simulink model "Simulation"  (R2023b)
settings: Solver=VariableStepAuto  StartTime=0.0  StopTime=2  RelTol=1e-3
InitFcn:
  | Tsc=0.0001;
  | Rs=0.0113929;
  | Rr=0.0197883;
  | Ls=0.007145;
  | Lr=0.007145;
  | Lm=0.007045;
  | w_c=100;
libraries: slpidlib x6, simulink x1, spspowerguiLib x1
(part 1 of 2)
settings Model: Creator=zugzh  LastModifiedBy=zugzh
settings DebuggingCC: IgnoredZcDiagnostic=none

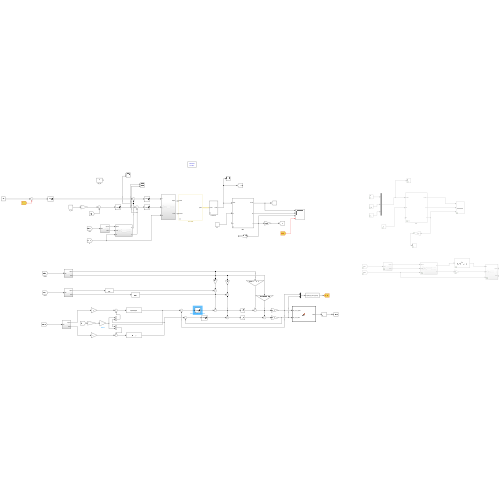
[thumbnail: Simulink's stored preview of the top-level diagram]
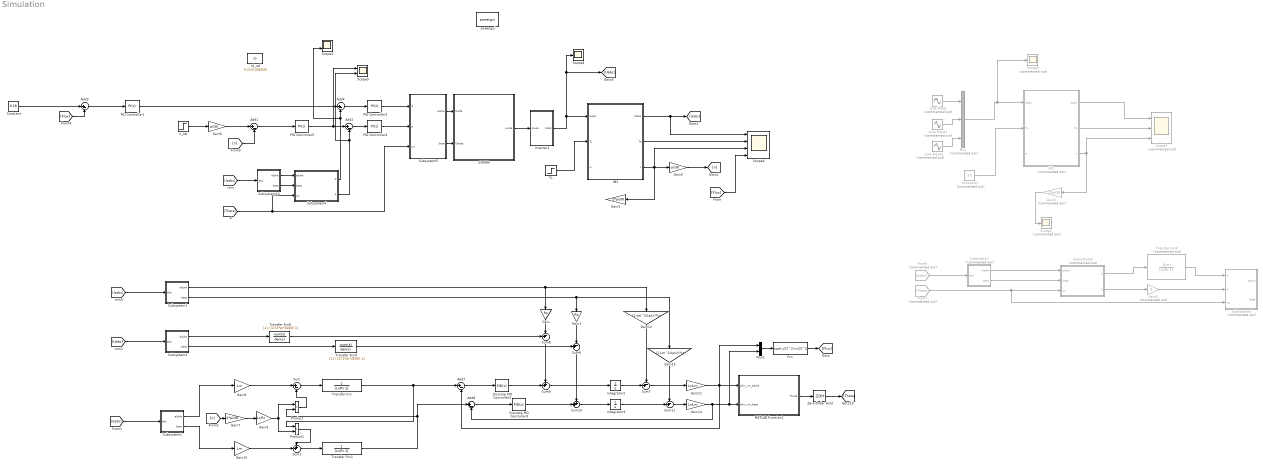
== system Simulation ==
  Add{1..4,7..8} (6 alike) : Sum  Inputs=|+-
  Constant : Constant  Value=0.18
  Constant1 : Constant  Commented=on  Value=75
  Discrete PID Controller2 : slpidlib/PID Controller  Controller=PID  Form=Parallel  TimeDomain=Discrete-time  UseExternalTs=off  SampleTime=-1  IntegratorMethod=Forward Euler  FilterMethod=Forward Euler  ControllerParametersSource=internal  P=sqrt(2)*w_c  I=w_c^2  UseKiTs=off  D=0  N=100  UseFilter=on  TunerSelectOption=Transfer Function Based (PID Tuner App)  InitialConditionSource=internal  InitialConditionForIntegrator=0  InitialConditionForFilter=0  DifferentiatorICPrevScaledInput=0  ExternalReset=none  TrackingMode=off  Kt=1  LimitOutput=on  SatLimitsSource=internal  UpperSaturationLimit=340  LowerSaturationLimit=-340  LinearizeAsGain=off  AntiWindupMode=none  Kb=1  LimitIntegrator=off  UpperIntegratorSaturationLimit=inf  LowerIntegratorSaturationLimit=-inf  POutMin=[]  POutMax=[]  IOutMin=[]  IOutMax=[]  DOutMin=[]  DOutMax=[]  NOutMin=[]  NOutMax=[]  SumOutMin=[]  SumOutMax=[]  SaturationOutMin=[]  SaturationOutMax=[]  PParamMin=[]  PParamMax=[]  IParamMin=[]  IParamMax=[]  DParamMin=[]  DParamMax=[]  NParamMin=[]  NParamMax=[]  KbParamMin=[]  KbParamMax=[]  KtParamMin=[]  KtParamMax=[]  KbOutMin=[]  KbOutMax=[]  KtOutMin=[]  KtOutMax=[]  IntegratorOutMin=[]  IntegratorOutMax=[]  FilterOutMin=[]  FilterOutMax=[]  SumI1OutMin=[]  SumI1OutMax=[]  SumI2OutMin=[]  SumI2OutMax=[]  SumI3OutMin=[]  SumI3OutMax=[]  SumI4OutMin=[]  SumI4OutMax=[]  SumDOutMin=[]  SumDOutMax=[]  DifferentiatorOutMin=[]  DifferentiatorOutMax=[]  FilterDiffOutCoefMin=[]  FilterDiffOutCoefMax=[]  ReciprocalOutMin=[]  ReciprocalOutMax=[]  SumDenOutMin=[]  SumDenOutMax=[]  SumNumOutMin=[]  SumNumOutMax=[]  DivideOutMin=[]  DivideOutMax=[]  UdiffTsProdOutMin=[]  UdiffTsProdOutMax=[]  NTsProdOutMin=[]  NTsProdOutMax=[]  UintegralTsProdOutMin=[]  UintegralTsProdOutMax=[]  UngainTsProdOutMin=[]  UngainTsProdOutMax=[]  ClampingZeroOutDataTypeStr=Inherit: Inherit via back propagation  ClampingZeroOutMin=[]  ClampingZeroOutMax=[]  FilterDenConstantOutDataTypeStr=Inherit: Inherit via back propagation  FilterDenConstantOutMin=[]  FilterDenConstantOutMax=[]  PCopyOutDataTypeStr=Inherit: Inherit via back propagation  PCopyOutMin=[]  PCopyOutMax=[]  NCopyOutDataTypeStr=Inherit: Inherit via back propagation  NCopyOutMin=[]  NCopyOutMax=[]  IntegratorContinuousStateAttributes=''  IntegratorStateMustResolveToSignalObject=off  IntegratorRTWStateStorageClass=Auto  FilterContinuousStateAttributes=''  FilterStateMustResolveToSignalObject=off  FilterRTWStateStorageClass=Auto  ParallelPVariant=InternalParameters  IdealPVariant=Disabled  IVariant=InternalParameters  DVariant=InternalParameters  IntegratorVariant=Discrete  SatVariant=Enabled  AWVariant=Passthrough  PCopyVariant=Disabled  TRVariant=Disabled  FdbkBlocksVariant=Forward  IdealPFdbkVariant=Disabled  SatFdbkVariant=Disabled  DerivativeFilterVariant=ForwardEulerFilter  NVariant=InternalParameters  NCopyVariant=Disabled  FilterICVariant=InternalICsFilter  IntegratorICVariant=InternalICs  ExternalResetVariant=Disabled  TRSumVariant=Passthrough  SumFdbkVariant=Disabled  SumVariant=Sum_PID  TsampFilterVariant=InternalTs  TsampNgainVariant=Passthrough  TsampIntegralVariant=Disabled_SignalSpec  ExternalSaturationOutDataTypeStr=Inherit: Same as second input
      settings: LibrarySourceBlock=hdlsllib/Discrete/Discrete PID Controller
  Discrete PID Controller3 : slpidlib/PID Controller  Controller=PID  Form=Parallel  TimeDomain=Discrete-time  UseExternalTs=off  SampleTime=-1  IntegratorMethod=Forward Euler  FilterMethod=Forward Euler  ControllerParametersSource=internal  P=sqrt(2)*w_c  I=w_c^2  UseKiTs=off  D=0  N=100  UseFilter=on  TunerSelectOption=Transfer Function Based (PID Tuner App)  InitialConditionSource=internal  InitialConditionForIntegrator=0  InitialConditionForFilter=0  DifferentiatorICPrevScaledInput=0  ExternalReset=none  TrackingMode=off  Kt=1  LimitOutput=on  SatLimitsSource=internal  UpperSaturationLimit=340  LowerSaturationLimit=-340  LinearizeAsGain=off  AntiWindupMode=none  Kb=1  LimitIntegrator=off  UpperIntegratorSaturationLimit=inf  LowerIntegratorSaturationLimit=-inf  POutMin=[]  POutMax=[]  IOutMin=[]  IOutMax=[]  DOutMin=[]  DOutMax=[]  NOutMin=[]  NOutMax=[]  SumOutMin=[]  SumOutMax=[]  SaturationOutMin=[]  SaturationOutMax=[]  PParamMin=[]  PParamMax=[]  IParamMin=[]  IParamMax=[]  DParamMin=[]  DParamMax=[]  NParamMin=[]  NParamMax=[]  KbParamMin=[]  KbParamMax=[]  KtParamMin=[]  KtParamMax=[]  KbOutMin=[]  KbOutMax=[]  KtOutMin=[]  KtOutMax=[]  IntegratorOutMin=[]  IntegratorOutMax=[]  FilterOutMin=[]  FilterOutMax=[]  SumI1OutMin=[]  SumI1OutMax=[]  SumI2OutMin=[]  SumI2OutMax=[]  SumI3OutMin=[]  SumI3OutMax=[]  SumI4OutMin=[]  SumI4OutMax=[]  SumDOutMin=[]  SumDOutMax=[]  DifferentiatorOutMin=[]  DifferentiatorOutMax=[]  FilterDiffOutCoefMin=[]  FilterDiffOutCoefMax=[]  ReciprocalOutMin=[]  ReciprocalOutMax=[]  SumDenOutMin=[]  SumDenOutMax=[]  SumNumOutMin=[]  SumNumOutMax=[]  DivideOutMin=[]  DivideOutMax=[]  UdiffTsProdOutMin=[]  UdiffTsProdOutMax=[]  NTsProdOutMin=[]  NTsProdOutMax=[]  UintegralTsProdOutMin=[]  UintegralTsProdOutMax=[]  UngainTsProdOutMin=[]  UngainTsProdOutMax=[]  ClampingZeroOutDataTypeStr=Inherit: Inherit via back propagation  ClampingZeroOutMin=[]  ClampingZeroOutMax=[]  FilterDenConstantOutDataTypeStr=Inherit: Inherit via back propagation  FilterDenConstantOutMin=[]  FilterDenConstantOutMax=[]  PCopyOutDataTypeStr=Inherit: Inherit via back propagation  PCopyOutMin=[]  PCopyOutMax=[]  NCopyOutDataTypeStr=Inherit: Inherit via back propagation  NCopyOutMin=[]  NCopyOutMax=[]  IntegratorContinuousStateAttributes=''  IntegratorStateMustResolveToSignalObject=off  IntegratorRTWStateStorageClass=Auto  FilterContinuousStateAttributes=''  FilterStateMustResolveToSignalObject=off  FilterRTWStateStorageClass=Auto  ParallelPVariant=InternalParameters  IdealPVariant=Disabled  IVariant=InternalParameters  DVariant=InternalParameters  IntegratorVariant=Discrete  SatVariant=Enabled  AWVariant=Passthrough  PCopyVariant=Disabled  TRVariant=Disabled  FdbkBlocksVariant=Forward  IdealPFdbkVariant=Disabled  SatFdbkVariant=Disabled  DerivativeFilterVariant=ForwardEulerFilter  NVariant=InternalParameters  NCopyVariant=Disabled  FilterICVariant=InternalICsFilter  IntegratorICVariant=InternalICs  ExternalResetVariant=Disabled  TRSumVariant=Passthrough  SumFdbkVariant=Disabled  SumVariant=Sum_PID  TsampFilterVariant=InternalTs  TsampNgainVariant=Passthrough  TsampIntegralVariant=Disabled_SignalSpec  ExternalSaturationOutDataTypeStr=Inherit: Same as second input
      settings: LibrarySourceBlock=hdlsllib/Discrete/Discrete PID Controller
  Fcn : Fcn  Expr=sqrt(u(1)^2+u(2)^2)
  From6 : From  Commented=on  GotoTag=Isabc
  From7 : From  Commented=on  GotoTag=Theta
  Gain : Gain  Gain=Rs
  Gain1 : Gain  Gain=Rs
  Gain10 : Gain  Gain=Lm
  Gain11 : Gain  Gain=Lr/Lm
  Gain12 : Gain  Gain=(1-Lm^2/Ls/Lr)*Ls
  Gain14 : Gain  Gain=Lr/Lm
  Gain15 : Gain  Gain=(1-Lm^2/Ls/Lr)*Ls
  Gain2 : Gain  Commented=on  Gain=2*pi/30
  Gain3 : Gain  Gain=2*pi/30
  Gain4 : Gain  Commented=on  Gain=0
  Gain5 : Gain  Gain=pi/30
  Gain6 : Gain  Gain=pi/30
  Gain7 : Gain  Gain=2*pi/30
  Gain8 : Gain  Gain=Lm
  Gain9 : Gain  Gain=Lr/Rr
  IM1 : Subsystem  Commented=on  mask{Rs=0.0113929, Rr=0.0197883, Ls=0.006145, Lr=0.006145, Lm=0.006045, J=0.0952384, np=2}
      mask prompts: Rs "Rs(Ohm)"; Rr "Rr(Ohm)"; Ls "Ls(H)"; Lr "Lr(H)"; Lm "Lm(H)"; J "J(kg*m^2)"; np "Np()"
  IM2 : Subsystem  mask{Rs=0.0113929, Rr=0.0197883, Ls=0.007145, Lr=0.007145, Lm=0.007045, J=0.0952384, np=2}
      mask prompts: Rs "Rs(Ohm)"; Rr "Rr(Ohm)"; Ls "Ls(H)"; Lr "Lr(H)"; Lm "Lm(H)"; J "J(kg*m^2)"; np "Np()"
  Id_ref : Constant  Value=0.21/0.006045
  Integrator2 : Integrator  InitialCondition=0.001  LimitOutput=on  UpperSaturationLimit=1e6  LowerSaturationLimit=-1e6
  Integrator3 : Integrator  InitialCondition=0.001  LimitOutput=on  UpperSaturationLimit=1e6  LowerSaturationLimit=-1e6
  Inverter1 : Subsystem  mask(Inverter){Udc=540}
      mask prompts: Udc "Udc(V)"
  MATLAB Function1 : MATLAB Function  TreatAsAtomicUnit=on
  Mux : Mux  Commented=on  Inputs=3
  Mux1 : Mux  Inputs=2
  PID Controller1 : slpidlib/PID Controller  Controller=PI  Form=Parallel  TimeDomain=Discrete-time  UseExternalTs=off  SampleTime=-1  IntegratorMethod=Forward Euler  FilterMethod=Forward Euler  ControllerParametersSource=internal  P=1000  I=4000  UseKiTs=off  D=1  N=100  UseFilter=on  TunerSelectOption=Transfer Function Based (PID Tuner App)  InitialConditionSource=internal  InitialConditionForIntegrator=0  InitialConditionForFilter=0  DifferentiatorICPrevScaledInput=0  ExternalReset=none  TrackingMode=off  Kt=1  LimitOutput=on  SatLimitsSource=internal  UpperSaturationLimit=340  LowerSaturationLimit=-340  LinearizeAsGain=on  AntiWindupMode=none  Kb=1  LimitIntegrator=off  UpperIntegratorSaturationLimit=inf  LowerIntegratorSaturationLimit=-inf  POutMin=[]  POutMax=[]  IOutMin=[]  IOutMax=[]  DOutMin=[]  DOutMax=[]  NOutMin=[]  NOutMax=[]  SumOutMin=[]  SumOutMax=[]  SaturationOutMin=[]  SaturationOutMax=[]  PParamMin=[]  PParamMax=[]  IParamMin=[]  IParamMax=[]  DParamMin=[]  DParamMax=[]  NParamMin=[]  NParamMax=[]  KbParamMin=[]  KbParamMax=[]  KtParamMin=[]  KtParamMax=[]  KbOutMin=[]  KbOutMax=[]  KtOutMin=[]  KtOutMax=[]  IntegratorOutMin=[]  IntegratorOutMax=[]  FilterOutMin=[]  FilterOutMax=[]  SumI1OutMin=[]  SumI1OutMax=[]  SumI2OutMin=[]  SumI2OutMax=[]  SumI3OutMin=[]  SumI3OutMax=[]  SumI4OutMin=[]  SumI4OutMax=[]  SumDOutMin=[]  SumDOutMax=[]  DifferentiatorOutMin=[]  DifferentiatorOutMax=[]  FilterDiffOutCoefMin=[]  FilterDiffOutCoefMax=[]  ReciprocalOutMin=[]  ReciprocalOutMax=[]  SumDenOutMin=[]  SumDenOutMax=[]  SumNumOutMin=[]  SumNumOutMax=[]  DivideOutMin=[]  DivideOutMax=[]  UdiffTsProdOutMin=[]  UdiffTsProdOutMax=[]  NTsProdOutMin=[]  NTsProdOutMax=[]  UintegralTsProdOutMin=[]  UintegralTsProdOutMax=[]  UngainTsProdOutMin=[]  UngainTsProdOutMax=[]  ClampingZeroOutDataTypeStr=Inherit: Inherit via back propagation  ClampingZeroOutMin=[]  ClampingZeroOutMax=[]  FilterDenConstantOutDataTypeStr=Inherit: Inherit via back propagation  FilterDenConstantOutMin=[]  FilterDenConstantOutMax=[]  PCopyOutDataTypeStr=Inherit: Inherit via back propagation  PCopyOutMin=[]  PCopyOutMax=[]  NCopyOutDataTypeStr=Inherit: Inherit via back propagation  NCopyOutMin=[]  NCopyOutMax=[]  IntegratorContinuousStateAttributes=''  IntegratorStateMustResolveToSignalObject=off  IntegratorRTWStateStorageClass=Auto  FilterContinuousStateAttributes=''  FilterStateMustResolveToSignalObject=off  FilterRTWStateStorageClass=Auto  ParallelPVariant=InternalParameters  IdealPVariant=Disabled  IVariant=InternalParameters  DVariant=Disabled  IntegratorVariant=Discrete  SatVariant=Enabled  AWVariant=Passthrough  PCopyVariant=Disabled  TRVariant=Disabled  FdbkBlocksVariant=Forward  IdealPFdbkVariant=Disabled  SatFdbkVariant=Disabled  DerivativeFilterVariant=Disabled  NVariant=Disabled  NCopyVariant=Disabled_SignalSpec  FilterICVariant=Disabled  IntegratorICVariant=InternalICs  ExternalResetVariant=Disabled  TRSumVariant=Passthrough  SumFdbkVariant=Disabled  SumVariant=Sum_PI  TsampFilterVariant=InternalTs  TsampNgainVariant=Passthrough  TsampIntegralVariant=Disabled_SignalSpec  ExternalSaturationOutDataTypeStr=Inherit: Same as second input
  PID Controller3 : slpidlib/PID Controller  Controller=PI  Form=Parallel  TimeDomain=Discrete-time  UseExternalTs=off  SampleTime=-1  IntegratorMethod=Forward Euler  FilterMethod=Forward Euler  ControllerParametersSource=internal  P=0.656736650875738  I=37.717571379892140  UseKiTs=off  D=1  N=100  UseFilter=on  TunerSelectOption=Transfer Function Based (PID Tuner App)  InitialConditionSource=internal  InitialConditionForIntegrator=0  InitialConditionForFilter=0  DifferentiatorICPrevScaledInput=0  ExternalReset=none  TrackingMode=off  Kt=1  LimitOutput=on  SatLimitsSource=internal  UpperSaturationLimit=340  LowerSaturationLimit=-340  LinearizeAsGain=on  AntiWindupMode=none  Kb=1  LimitIntegrator=off  UpperIntegratorSaturationLimit=inf  LowerIntegratorSaturationLimit=-inf  POutMin=[]  POutMax=[]  IOutMin=[]  IOutMax=[]  DOutMin=[]  DOutMax=[]  NOutMin=[]  NOutMax=[]  SumOutMin=[]  SumOutMax=[]  SaturationOutMin=[]  SaturationOutMax=[]  PParamMin=[]  PParamMax=[]  IParamMin=[]  IParamMax=[]  DParamMin=[]  DParamMax=[]  NParamMin=[]  NParamMax=[]  KbParamMin=[]  KbParamMax=[]  KtParamMin=[]  KtParamMax=[]  KbOutMin=[]  KbOutMax=[]  KtOutMin=[]  KtOutMax=[]  IntegratorOutMin=[]  IntegratorOutMax=[]  FilterOutMin=[]  FilterOutMax=[]  SumI1OutMin=[]  SumI1OutMax=[]  SumI2OutMin=[]  SumI2OutMax=[]  SumI3OutMin=[]  SumI3OutMax=[]  SumI4OutMin=[]  SumI4OutMax=[]  SumDOutMin=[]  SumDOutMax=[]  DifferentiatorOutMin=[]  DifferentiatorOutMax=[]  FilterDiffOutCoefMin=[]  FilterDiffOutCoefMax=[]  ReciprocalOutMin=[]  ReciprocalOutMax=[]  SumDenOutMin=[]  SumDenOutMax=[]  SumNumOutMin=[]  SumNumOutMax=[]  DivideOutMin=[]  DivideOutMax=[]  UdiffTsProdOutMin=[]  UdiffTsProdOutMax=[]  NTsProdOutMin=[]  NTsProdOutMax=[]  UintegralTsProdOutMin=[]  UintegralTsProdOutMax=[]  UngainTsProdOutMin=[]  UngainTsProdOutMax=[]  ClampingZeroOutDataTypeStr=Inherit: Inherit via back propagation  ClampingZeroOutMin=[]  ClampingZeroOutMax=[]  FilterDenConstantOutDataTypeStr=Inherit: Inherit via back propagation  FilterDenConstantOutMin=[]  FilterDenConstantOutMax=[]  PCopyOutDataTypeStr=Inherit: Inherit via back propagation  PCopyOutMin=[]  PCopyOutMax=[]  NCopyOutDataTypeStr=Inherit: Inherit via back propagation  NCopyOutMin=[]  NCopyOutMax=[]  IntegratorContinuousStateAttributes=''  IntegratorStateMustResolveToSignalObject=off  IntegratorRTWStateStorageClass=Auto  FilterContinuousStateAttributes=''  FilterStateMustResolveToSignalObject=off  FilterRTWStateStorageClass=Auto  ParallelPVariant=InternalParameters  IdealPVariant=Disabled  IVariant=InternalParameters  DVariant=Disabled  IntegratorVariant=Discrete  SatVariant=Enabled  AWVariant=Passthrough  PCopyVariant=Disabled  TRVariant=Disabled  FdbkBlocksVariant=Forward  IdealPFdbkVariant=Disabled  SatFdbkVariant=Disabled  DerivativeFilterVariant=Disabled  NVariant=Disabled  NCopyVariant=Disabled_SignalSpec  FilterICVariant=Disabled  IntegratorICVariant=InternalICs  ExternalResetVariant=Disabled  TRSumVariant=Passthrough  SumFdbkVariant=Disabled  SumVariant=Sum_PI  TsampFilterVariant=InternalTs  TsampNgainVariant=Passthrough  TsampIntegralVariant=Disabled_SignalSpec  ExternalSaturationOutDataTypeStr=Inherit: Same as second input
  PID Controller4 : slpidlib/PID Controller  Controller=PI  Form=Parallel  TimeDomain=Discrete-time  UseExternalTs=off  SampleTime=-1  IntegratorMethod=Forward Euler  FilterMethod=Forward Euler  ControllerParametersSource=internal  P=0.656736650875738  I=1.011142867406485e+02  UseKiTs=off  D=1  N=100  UseFilter=on  TunerSelectOption=Transfer Function Based (PID Tuner App)  InitialConditionSource=internal  InitialConditionForIntegrator=0  InitialConditionForFilter=0  DifferentiatorICPrevScaledInput=0  ExternalReset=none  TrackingMode=off  Kt=1  LimitOutput=on  SatLimitsSource=internal  UpperSaturationLimit=340  LowerSaturationLimit=-340  LinearizeAsGain=on  AntiWindupMode=none  Kb=1  LimitIntegrator=off  UpperIntegratorSaturationLimit=inf  LowerIntegratorSaturationLimit=-inf  POutMin=[]  POutMax=[]  IOutMin=[]  IOutMax=[]  DOutMin=[]  DOutMax=[]  NOutMin=[]  NOutMax=[]  SumOutMin=[]  SumOutMax=[]  SaturationOutMin=[]  SaturationOutMax=[]  PParamMin=[]  PParamMax=[]  IParamMin=[]  IParamMax=[]  DParamMin=[]  DParamMax=[]  NParamMin=[]  NParamMax=[]  KbParamMin=[]  KbParamMax=[]  KtParamMin=[]  KtParamMax=[]  KbOutMin=[]  KbOutMax=[]  KtOutMin=[]  KtOutMax=[]  IntegratorOutMin=[]  IntegratorOutMax=[]  FilterOutMin=[]  FilterOutMax=[]  SumI1OutMin=[]  SumI1OutMax=[]  SumI2OutMin=[]  SumI2OutMax=[]  SumI3OutMin=[]  SumI3OutMax=[]  SumI4OutMin=[]  SumI4OutMax=[]  SumDOutMin=[]  SumDOutMax=[]  DifferentiatorOutMin=[]  DifferentiatorOutMax=[]  FilterDiffOutCoefMin=[]  FilterDiffOutCoefMax=[]  ReciprocalOutMin=[]  ReciprocalOutMax=[]  SumDenOutMin=[]  SumDenOutMax=[]  SumNumOutMin=[]  SumNumOutMax=[]  DivideOutMin=[]  DivideOutMax=[]  UdiffTsProdOutMin=[]  UdiffTsProdOutMax=[]  NTsProdOutMin=[]  NTsProdOutMax=[]  UintegralTsProdOutMin=[]  UintegralTsProdOutMax=[]  UngainTsProdOutMin=[]  UngainTsProdOutMax=[]  ClampingZeroOutDataTypeStr=Inherit: Inherit via back propagation  ClampingZeroOutMin=[]  ClampingZeroOutMax=[]  FilterDenConstantOutDataTypeStr=Inherit: Inherit via back propagation  FilterDenConstantOutMin=[]  FilterDenConstantOutMax=[]  PCopyOutDataTypeStr=Inherit: Inherit via back propagation  PCopyOutMin=[]  PCopyOutMax=[]  NCopyOutDataTypeStr=Inherit: Inherit via back propagation  NCopyOutMin=[]  NCopyOutMax=[]  IntegratorContinuousStateAttributes=''  IntegratorStateMustResolveToSignalObject=off  IntegratorRTWStateStorageClass=Auto  FilterContinuousStateAttributes=''  FilterStateMustResolveToSignalObject=off  FilterRTWStateStorageClass=Auto  ParallelPVariant=InternalParameters  IdealPVariant=Disabled  IVariant=InternalParameters  DVariant=Disabled  IntegratorVariant=Discrete  SatVariant=Enabled  AWVariant=Passthrough  PCopyVariant=Disabled  TRVariant=Disabled  FdbkBlocksVariant=Forward  IdealPFdbkVariant=Disabled  SatFdbkVariant=Disabled  DerivativeFilterVariant=Disabled  NVariant=Disabled  NCopyVariant=Disabled_SignalSpec  FilterICVariant=Disabled  IntegratorICVariant=InternalICs  ExternalResetVariant=Disabled  TRSumVariant=Passthrough  SumFdbkVariant=Disabled  SumVariant=Sum_PI  TsampFilterVariant=InternalTs  TsampNgainVariant=Passthrough  TsampIntegralVariant=Disabled_SignalSpec  ExternalSaturationOutDataTypeStr=Inherit: Same as second input
  PID Controller5 : slpidlib/PID Controller  Controller=PI  Form=Parallel  TimeDomain=Discrete-time  UseExternalTs=off  SampleTime=Tsc  IntegratorMethod=Forward Euler  FilterMethod=Forward Euler  ControllerParametersSource=internal  P=2.769062140173488e+03  I=1.980890752650220e+06  UseKiTs=off  D=0  N=100  UseFilter=on  TunerSelectOption=Transfer Function Based (PID Tuner App)  InitialConditionSource=internal  InitialConditionForIntegrator=0  InitialConditionForFilter=0  DifferentiatorICPrevScaledInput=0  ExternalReset=none  TrackingMode=off  Kt=1  LimitOutput=on  SatLimitsSource=internal  UpperSaturationLimit=196  LowerSaturationLimit=-196  LinearizeAsGain=off  AntiWindupMode=clamping  Kb=1  LimitIntegrator=off  UpperIntegratorSaturationLimit=inf  LowerIntegratorSaturationLimit=-inf  POutMin=[]  POutMax=[]  IOutMin=[]  IOutMax=[]  DOutMin=[]  DOutMax=[]  NOutMin=[]  NOutMax=[]  SumOutMin=[]  SumOutMax=[]  SaturationOutMin=[]  SaturationOutMax=[]  PParamMin=[]  PParamMax=[]  IParamMin=[]  IParamMax=[]  DParamMin=[]  DParamMax=[]  NParamMin=[]  NParamMax=[]  KbParamMin=[]  KbParamMax=[]  KtParamMin=[]  KtParamMax=[]  KbOutMin=[]  KbOutMax=[]  KtOutMin=[]  KtOutMax=[]  IntegratorOutMin=[]  IntegratorOutMax=[]  FilterOutMin=[]  FilterOutMax=[]  SumI1OutMin=[]  SumI1OutMax=[]  SumI2OutMin=[]  SumI2OutMax=[]  SumI3OutMin=[]  SumI3OutMax=[]  SumI4OutMin=[]  SumI4OutMax=[]  SumDOutMin=[]  SumDOutMax=[]  DifferentiatorOutMin=[]  DifferentiatorOutMax=[]  FilterDiffOutCoefMin=[]  FilterDiffOutCoefMax=[]  ReciprocalOutMin=[]  ReciprocalOutMax=[]  SumDenOutMin=[]  SumDenOutMax=[]  SumNumOutMin=[]  SumNumOutMax=[]  DivideOutMin=[]  DivideOutMax=[]  UdiffTsProdOutMin=[]  UdiffTsProdOutMax=[]  NTsProdOutMin=[]  NTsProdOutMax=[]  UintegralTsProdOutMin=[]  UintegralTsProdOutMax=[]  UngainTsProdOutMin=[]  UngainTsProdOutMax=[]  ClampingZeroOutDataTypeStr=Inherit: Inherit via back propagation  ClampingZeroOutMin=[]  ClampingZeroOutMax=[]  FilterDenConstantOutDataTypeStr=Inherit: Inherit via back propagation  FilterDenConstantOutMin=[]  FilterDenConstantOutMax=[]  PCopyOutDataTypeStr=Inherit: Inherit via back propagation  PCopyOutMin=[]  PCopyOutMax=[]  NCopyOutDataTypeStr=Inherit: Inherit via back propagation  NCopyOutMin=[]  NCopyOutMax=[]  IntegratorContinuousStateAttributes=''  IntegratorStateMustResolveToSignalObject=off  IntegratorRTWStateStorageClass=Auto  FilterContinuousStateAttributes=''  FilterStateMustResolveToSignalObject=off  FilterRTWStateStorageClass=Auto  ParallelPVariant=InternalParameters  IdealPVariant=Disabled  IVariant=InternalParameters  DVariant=Disabled  IntegratorVariant=Discrete  SatVariant=Enabled  AWVariant=DiscClampingParallel  PCopyVariant=Disabled  TRVariant=Disabled  FdbkBlocksVariant=Forward  IdealPFdbkVariant=Disabled  SatFdbkVariant=Disabled  DerivativeFilterVariant=Disabled  NVariant=Disabled  NCopyVariant=Disabled_SignalSpec  FilterICVariant=Disabled  IntegratorICVariant=InternalICs  ExternalResetVariant=Disabled  TRSumVariant=Passthrough  SumFdbkVariant=Disabled  SumVariant=Sum_PI  TsampFilterVariant=InternalTs  TsampNgainVariant=Passthrough  TsampIntegralVariant=Disabled_SignalSpec  ExternalSaturationOutDataTypeStr=Inherit: Same as second input
  Product : Product
  Product1 : Product
  SVPWM : Subsystem  mask{Ts=1/10000, Udc=540}
  Scope1 : Scope  Commented=on
  Scope2 : Scope  NumInputPorts=2
  Scope3 : Scope  Commented=on  NumInputPorts=3
  Scope4 : Scope  NumInputPorts=4
  Scope5 : Scope  NumInputPorts=2
  Scope8 : Scope
  Scope9 : Scope  Commented=on
  Sine Wave : Sin  Commented=on  Amplitude=244.949  Frequency=4567.25/60*2*2*pi*(1+0.0425049)  SampleTime=0
  Sine Wave1 : Sin  Commented=on  Amplitude=244.949  Frequency=4567.25/60*2*2*pi*(1+0.0425049)  Phase=-2*pi/3  SampleTime=0
  Sine Wave2 : Sin  Commented=on  Amplitude=244.949  Frequency=4567.25/60*2*2*pi*(1+0.0425049)  Phase=-4*pi/3  SampleTime=0
  Subsystem1 : Subsystem
  Subsystem10 : Subsystem
  Subsystem2 : Subsystem
  Subsystem3 : Subsystem
  Subsystem4 : Subsystem
  Subsystem5 : Subsystem
  Subsystem6 : Subsystem  Commented=on
  Subsystem7 : Subsystem  Commented=on
  Subsystem8 : Subsystem  Commented=on
  Sum : Sum  Inputs=|+-
  Sum1 : Sum  Inputs=++|
  Sum10 : Sum  Inputs=++|
  Sum11 : Sum  Inputs=-+|
  Sum6 : Sum  Inputs=+-|
  Sum7 : Sum  Inputs=-+|
  Sum8 : Sum  Inputs=+-|
  Sum9 : Sum  Inputs=++|
  TL : Step  After=0  SampleTime=Tsc
  Transfer Fcn : TransferFcn  Denominator=[Lr/Rr 1]
  Transfer Fcn1 : TransferFcn  Denominator=[Lr/Rr 1]
  Transfer Fcn3 : TransferFcn  Commented=on  Numerator=[Lm]  Denominator=[Lr/Rr 1]
  Transfer Fcn8 : TransferFcn  Denominator=[1/(2*pi*4000) 1]
  Transfer Fcn9 : TransferFcn  Denominator=[1/(2*pi*4000) 1]
  Zero-Order Hold : ZeroOrderHold  SampleTime=-1
  n_ref : Step  Time=1.4  Before=50  After=50  SampleTime=Tsc
  powergui : spspowerguiLib/powergui  Priority=1  SimulationMode=Discrete  SampleTime=1e-5  frequency=60  Iterations=50  frequencyindice=0  Pbase=100e6  ErrMax=1e-4  UnitsV=kV  UnitsW=MW  buscounter=0  FunctionMessages=off  echomessages=off  EnableUseOfTLC=off  CurrentSourceSwitches=off  DisableSnubberDevices=off  DisableRonSwitches=off  DisableVfSwitches=off  DisplayEquations=off  AutomaticDiscreteSolvers=off  SolverType=Tustin/Backward Euler (TBE)  Interpol=off  ExternalGateDelay=off  methode=off  Ts=10  x0status=blocks  SPID=off  SwTol=0  HookPort=off  NonlinearTolerance=1e-4  nMaxIteration=100  ContinueOnMaxIteration=off  RestoreLinks=warning  ResistiveCurrentMeasurement=off  Frange=[0:2:500]  Ylog=off  Xlog=on  ShowGrid=off  save=off  variable=ZData  structure=ScopeData3  ZoomFFT=off  StartTime=0.01  cycles=2  DisplayStyle=1  fundamental=50  FreqAxis=off  MaxFrequency=25000  frequencyindicesteady=1  RmsSteady=1  display=off
  wires:
  Sine Wave/1 -> Mux/1
  Sine Wave1/1 -> Mux/2
  Sine Wave2/1 -> Mux/3
  Mux/1 -> Scope9/1, IM1/1(Uabc)
  IM1/1(Isabc) -> Scope3/1
  IM1/3(n) -> Scope3/3, Gain2/1
  Gain2/1 -> Scope1/1
  IM1/2(Te) -> Scope3/2
  IM2/2(Te) -> Scope4/2
  MATLAB Function1/1(Theta) -> Zero-Order Hold/1
  Integrator2/1 -> Sum7/2
  From7/1 -> Subsystem8/3(wt), Subsystem6/3(wt)
  Gain1/1 -> Sum6/2
  Sum8/1 -> Sum9/1
  Gain11/1 -> Add7/2, Mux1/1, MATLAB Function1/1(phir_vm_alpha)
  Zero-Order Hold/1 -> [Theta]
  Sum10/1 -> Integrator3/1
  Subsystem6/1(d) -> Transfer Fcn3/1
  Gain14/1 -> Mux1/2, MATLAB Function1/2(phir_vm_beta), Add8/2
  Add7/1 -> Discrete PID Controller2/1
  Gain/1 -> Sum8/2
  Discrete PID Controller3/1 -> Sum10/2
  Transfer Fcn3/1 -> Subsystem8/1(d)
  Gain12/1 -> Sum7/1
  Gain4/1 -> Subsystem8/2(q)
  Add8/1 -> Discrete PID Controller3/1
  Sum11/1 -> Gain14/1
  Sum6/1 -> Sum10/1
  Integrator3/1 -> Sum11/2
  Gain15/1 -> Sum11/1
  [Isabc] -> Subsystem1/1(abc)
  Discrete PID Controller2/1 -> Sum9/2
  Sum9/1 -> Integrator2/1
  Subsystem6/2(q) -> Gain4/1
  From6/1 -> Subsystem7/1(abc)
  Sum7/1 -> Gain11/1
  IM2/1(Isabc) -> Scope4/1, [Isabc]
  Subsystem1/1(alpha) -> Gain12/1, Gain/1
  Subsystem1/2(beta) -> Gain15/1, Gain1/1
  Subsystem7/1(alpha) -> Subsystem6/1(alpha)
  Subsystem7/2(beta) -> Subsystem6/2(beta)
  Inverter1/1(Uabc) -> IM2/1(Uabc), [Uabc], Scope8/1
  TL/1 -> IM2/2(TL)
  Constant1/1 -> IM1/2(TL)
  IM2/3(n) -> Scope4/3, Gain3/1, Gain5/1
  Transfer Fcn8/1 -> Sum8/1
  Transfer Fcn9/1 -> Sum6/1
  [Uabc] -> Subsystem3/1(abc)
  Subsystem3/1(alpha) -> Transfer Fcn8/1
  Subsystem3/2(beta) -> Transfer Fcn9/1
  Gain5/1 -> [n]
  [Flux] -> Scope4/4
  Subsystem5/2(beta) -> SVPWM/2(Ubeta)
  Subsystem5/1(alpha) -> SVPWM/1(Ualfa)
  [n] -> Add1/2
  [Theta] -> Subsystem4/3(wt), Subsystem5/3(wt)
  SVPWM/1(pulse) -> Inverter1/1(pluse)
  n_ref/1 -> Gain6/1
  Subsystem10/1(alpha) -> Subsystem4/1(alpha)
  Subsystem10/2(beta) -> Subsystem4/2(beta)
  [Isabc] -> Subsystem10/1(abc)
  Subsystem4/1(d) -> Scope2/2, Add4/2
  Subsystem4/2(q) -> Scope5/2, Add2/2
  Add4/1 -> PID Controller3/1
  PID Controller3/1 -> Subsystem5/1(d)
  Add2/1 -> PID Controller4/1
  PID Controller4/1 -> Subsystem5/2(q)
  Add1/1 -> PID Controller5/1
  PID Controller5/1 -> Scope5/1, Add2/1
  Gain6/1 -> Add1/1
  [Isabc] -> Subsystem2/1(abc)
  [n] -> Gain7/1
  Subsystem2/1(alpha) -> Gain8/1
  Subsystem2/2(beta) -> Gain10/1
  Gain8/1 -> Sum/1
  Gain7/1 -> Gain9/1
  Gain10/1 -> Sum1/2
  Sum1/1 -> Transfer Fcn1/1
  Sum/1 -> Transfer Fcn/1
  Transfer Fcn1/1 -> Add8/1, Product/2
  Gain9/1 -> Product/1, Product1/2
  Product/1 -> Sum/2
  Transfer Fcn/1 -> Add7/1, Product1/1
  Product1/1 -> Sum1/1
  Mux1/1 -> Fcn/1
  Fcn/1 -> [Flux]
  Add3/1 -> PID Controller1/1
  Constant/1 -> Add3/1
  [Flux] -> Add3/2
  PID Controller1/1 -> Add4/1

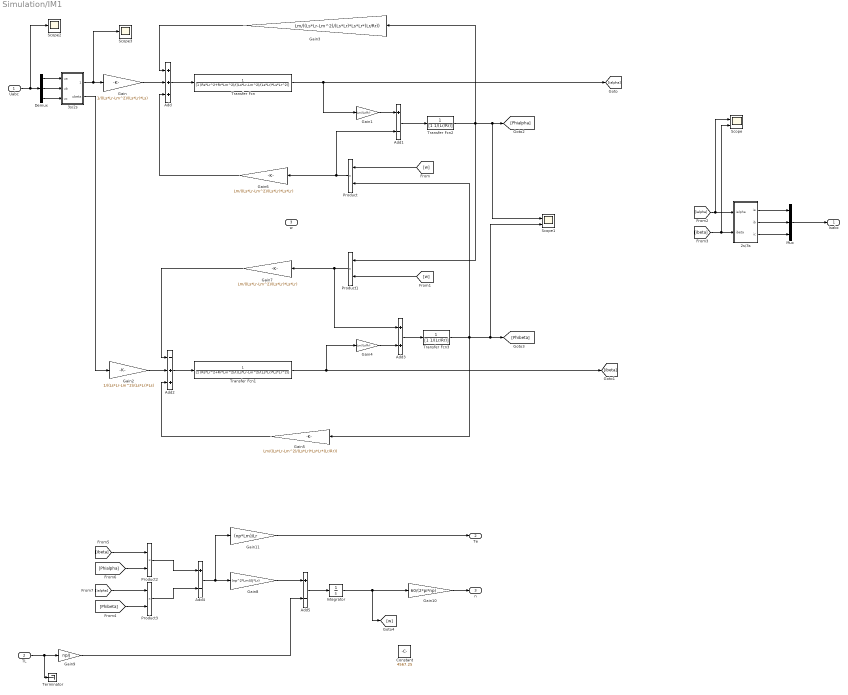
== system Simulation/IM1 ==
  Uabc : Inport
  TL : Inport  Port=2
  w : Inport  Port=3
  2s/3s : Subsystem
  3s/2s : Subsystem
  Add : Sum  Inputs=+++
  Add1 : Sum  Inputs=+-
  Add2 : Sum  Inputs=-++
  Add3 : Sum
  Add4 : Sum  Inputs=+-
  Add5 : Sum  Inputs=+-
  Constant : Constant  Value=4567.25
  Demux : Demux  Outputs=3
  Gain : Gain  Gain=1/((Ls*Lr-Lm^2)/(Ls*Lr)*Ls)
  Gain1 : Gain  Gain=Lm/(Lr/Rr)
  Gain10 : Gain  Gain=60/(2*pi*np)  SaturateOnIntegerOverflow=on  OutDataTypeStr=Inherit: Same as input  ParamDataTypeStr=Inherit: Same as input
  Gain11 : Gain  Gain=(np*Lm)/Lr
  Gain2 : Gain  Gain=1/((Ls*Lr-Lm^2)/(Ls*Lr)*Ls)
  Gain3 : Gain  Gain=Lm/((Ls*Lr-Lm^2)/(Ls*Lr)*Ls*Lr*(Lr/Rr))
  Gain4 : Gain  Gain=Lm/(Lr/Rr)
  Gain5 : Gain  Gain=Lm/((Ls*Lr-Lm^2)/(Ls*Lr)*Ls*Lr*(Lr/Rr))
  Gain6 : Gain  Gain=Lm/((Ls*Lr-Lm^2)/(Ls*Lr)*Ls*Lr)
  Gain7 : Gain  Gain=Lm/((Ls*Lr-Lm^2)/(Ls*Lr)*Ls*Lr)
  Gain8 : Gain  Gain=(np^2*Lm)/(J*Lr)
  Gain9 : Gain  Gain=np/J
  Integrator : Integrator
  Mux : Mux  Inputs=3
  Product{,1..3} (4 alike) : Product
  Scope : Scope  NumInputPorts=2
  Scope1 : Scope  NumInputPorts=2
  Scope2 : Scope
  Scope3 : Scope
  Terminator : Terminator
  Transfer Fcn : TransferFcn  Denominator=[1 (Rs*Lr^2+Rr*Lm^2)/((Ls*Lr-Lm^2)/(Ls*Lr)*Ls*Lr^2)]
  Transfer Fcn1 : TransferFcn  Denominator=[1 (Rs*Lr^2+Rr*Lm^2)/((Ls*Lr-Lm^2)/(Ls*Lr)*Ls*Lr^2)]
  Transfer Fcn2 : TransferFcn  Denominator=[1 1/(Lr/Rr)]
  Transfer Fcn3 : TransferFcn  Denominator=[1 1/(Lr/Rr)]
  Isabc : Outport
  Te : Outport  Port=2
  n : Outport  Port=3
  wires:
  Uabc/1 -> Scope2/1, Demux/1
  Demux/1 -> 3s/2s/1(ua)
  Demux/2 -> 3s/2s/2(ub)
  Demux/3 -> 3s/2s/3(uc)
  3s/2s/1(ualpha) -> Scope3/1, Gain/1
  Gain/1 -> Add/2
  Add/1 -> Transfer Fcn/1
  2s/3s/1(ia) -> Mux/1
  2s/3s/2(ib) -> Mux/2
  2s/3s/3(ic) -> Mux/3
  Transfer Fcn/1 -> [ialpha], Gain1/1
  Gain1/1 -> Add1/1
  Product/1 -> Add1/2, Gain6/1
  3s/2s/2(ubeta) -> Gain2/1
  Gain2/1 -> Add2/2
  Add2/1 -> Transfer Fcn1/1
  Transfer Fcn1/1 -> [ibeta], Gain4/1
  Add1/1 -> Transfer Fcn2/1
  Transfer Fcn2/1 -> Scope1/1, [Phialpha], Gain3/1, Product1/1
  Gain3/1 -> Add/1
  Gain4/1 -> Add3/2
  Add3/1 -> Transfer Fcn3/1
  Transfer Fcn3/1 -> Gain5/1, Scope1/2, [Phibeta], Product/2
  Gain5/1 -> Add2/3
  Gain6/1 -> Add/3
  Product1/1 -> Add3/1, Gain7/1
  Gain7/1 -> Add2/1
  Mux/1 -> Isabc/1
  [ialpha] -> Scope/1, 2s/3s/1(ialpha)
  [ibeta] -> Scope/2, 2s/3s/2(ibeta)
  [ibeta] -> Product2/1
  [Phialpha] -> Product2/2
  [ialpha] -> Product3/1
  [Phibeta] -> Product3/2
  Product2/1 -> Add4/1
  Product3/1 -> Add4/2
  Add4/1 -> Gain8/1, Gain11/1
  Gain8/1 -> Add5/1
  Gain9/1 -> Add5/2
  Add5/1 -> Integrator/1
  Integrator/1 -> Gain10/1, [w]
  Gain11/1 -> Te/1
  TL/1 -> Terminator/1, Gain9/1
  Gain10/1 -> n/1
  [w] -> Product/1
  [w] -> Product1/2

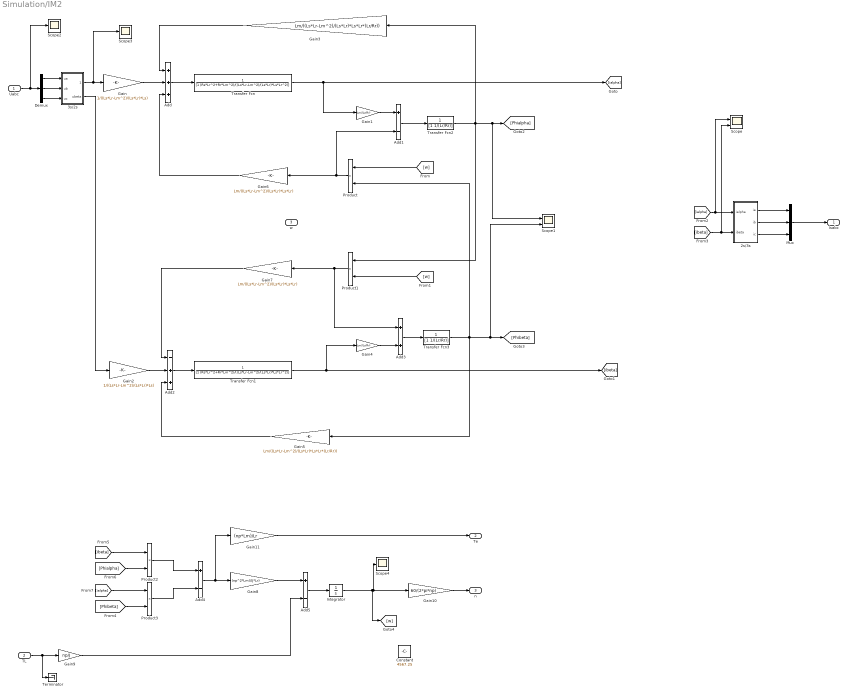
== system Simulation/IM2 ==
  Uabc : Inport
  TL : Inport  Port=2
  w : Inport  Port=3
  2s/3s : Subsystem
  3s/2s : Subsystem
  Add : Sum  Inputs=+++
  Add1 : Sum  Inputs=+-
  Add2 : Sum  Inputs=-++
  Add3 : Sum
  Add4 : Sum  Inputs=+-
  Add5 : Sum  Inputs=+-
  Constant : Constant  Value=4567.25
  Demux : Demux  Outputs=3
  Gain : Gain  Gain=1/((Ls*Lr-Lm^2)/(Ls*Lr)*Ls)
  Gain1 : Gain  Gain=Lm/(Lr/Rr)
  Gain10 : Gain  Gain=60/(2*pi*np)  SaturateOnIntegerOverflow=on  OutDataTypeStr=Inherit: Same as input  ParamDataTypeStr=Inherit: Same as input
  Gain11 : Gain  Gain=(np*Lm)/Lr
  Gain2 : Gain  Gain=1/((Ls*Lr-Lm^2)/(Ls*Lr)*Ls)
  Gain3 : Gain  Gain=Lm/((Ls*Lr-Lm^2)/(Ls*Lr)*Ls*Lr*(Lr/Rr))
  Gain4 : Gain  Gain=Lm/(Lr/Rr)
  Gain5 : Gain  Gain=Lm/((Ls*Lr-Lm^2)/(Ls*Lr)*Ls*Lr*(Lr/Rr))
  Gain6 : Gain  Gain=Lm/((Ls*Lr-Lm^2)/(Ls*Lr)*Ls*Lr)
  Gain7 : Gain  Gain=Lm/((Ls*Lr-Lm^2)/(Ls*Lr)*Ls*Lr)
  Gain8 : Gain  Gain=(np^2*Lm)/(J*Lr)
  Gain9 : Gain  Gain=np/J
  Integrator : Integrator  InitialCondition=0.001
  Mux : Mux  Inputs=3
  Product{,1..3} (4 alike) : Product
  Scope : Scope  NumInputPorts=2
  Scope1 : Scope  NumInputPorts=2
  Scope2 : Scope
  Scope3 : Scope
  Scope4 : Scope
  Terminator : Terminator
  Transfer Fcn : TransferFcn  Denominator=[1 (Rs*Lr^2+Rr*Lm^2)/((Ls*Lr-Lm^2)/(Ls*Lr)*Ls*Lr^2)]
  Transfer Fcn1 : TransferFcn  Denominator=[1 (Rs*Lr^2+Rr*Lm^2)/((Ls*Lr-Lm^2)/(Ls*Lr)*Ls*Lr^2)]
  Transfer Fcn2 : TransferFcn  Denominator=[1 1/(Lr/Rr)]
  Transfer Fcn3 : TransferFcn  Denominator=[1 1/(Lr/Rr)]
  Isabc : Outport
  Te : Outport  Port=2
  n : Outport  Port=3
  wires:
  Uabc/1 -> Scope2/1, Demux/1
  Demux/1 -> 3s/2s/1(ua)
  Demux/2 -> 3s/2s/2(ub)
  Demux/3 -> 3s/2s/3(uc)
  3s/2s/1(ualpha) -> Scope3/1, Gain/1
  Gain/1 -> Add/2
  Add/1 -> Transfer Fcn/1
  2s/3s/1(ia) -> Mux/1
  2s/3s/2(ib) -> Mux/2
  2s/3s/3(ic) -> Mux/3
  Transfer Fcn/1 -> [ialpha], Gain1/1
  Gain1/1 -> Add1/1
  Product/1 -> Add1/2, Gain6/1
  3s/2s/2(ubeta) -> Gain2/1
  Gain2/1 -> Add2/2
  Add2/1 -> Transfer Fcn1/1
  Transfer Fcn1/1 -> [ibeta], Gain4/1
  Add1/1 -> Transfer Fcn2/1
  Transfer Fcn2/1 -> Scope1/1, [Phialpha], Gain3/1, Product1/1
  Gain3/1 -> Add/1
  Gain4/1 -> Add3/2
  Add3/1 -> Transfer Fcn3/1
  Transfer Fcn3/1 -> Gain5/1, Scope1/2, [Phibeta], Product/2
  Gain5/1 -> Add2/3
  Gain6/1 -> Add/3
  Product1/1 -> Add3/1, Gain7/1
  Gain7/1 -> Add2/1
  Mux/1 -> Isabc/1
  [ialpha] -> Scope/1, 2s/3s/1(ialpha)
  [ibeta] -> Scope/2, 2s/3s/2(ibeta)
  [ibeta] -> Product2/1
  [Phialpha] -> Product2/2
  [ialpha] -> Product3/1
  [Phibeta] -> Product3/2
  Product2/1 -> Add4/1
  Product3/1 -> Add4/2
  Add4/1 -> Gain8/1, Gain11/1
  Gain8/1 -> Add5/1
  Gain9/1 -> Add5/2
  Add5/1 -> Integrator/1
  Integrator/1 -> Scope4/1, Gain10/1, [w]
  Gain11/1 -> Te/1
  TL/1 -> Terminator/1, Gain9/1
  [w] -> Product/1
  [w] -> Product1/2
  Gain10/1 -> n/1

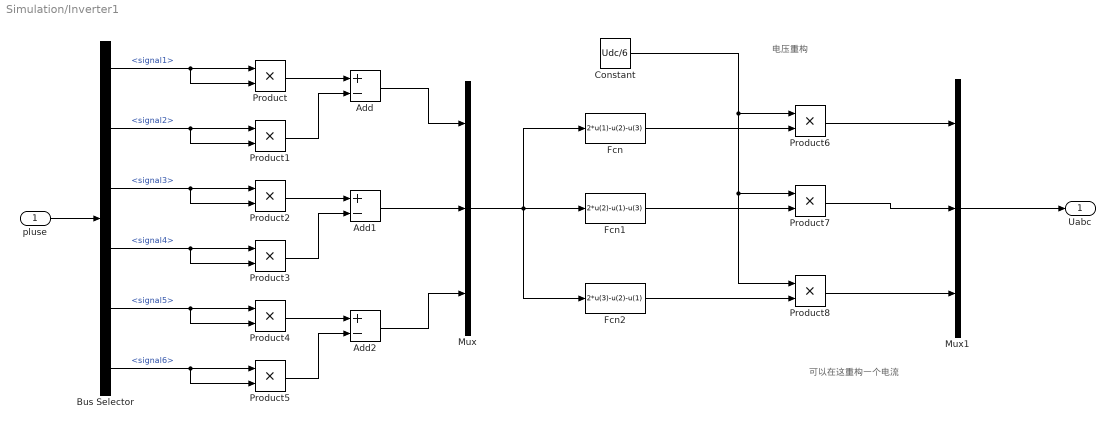
== system Simulation/Inverter1 ==
  note: 可以在这重构一个电流
  note: 电压重构
  pluse : Inport
  Add : Sum  Inputs=+-
  Add1 : Sum  Inputs=+-
  Add2 : Sum  Inputs=+-
  Bus Selector : BusSelector  OutputSignals=signal1,signal2,signal3,signal4,signal5,signal6
  Constant : Constant  Value=Udc/6
  Fcn : Fcn  Expr=2*u(1)-u(2)-u(3)
  Fcn1 : Fcn  Expr=2*u(2)-u(1)-u(3)
  Fcn2 : Fcn  Expr=2*u(3)-u(2)-u(1)
  Mux : Mux  Inputs=3
  Mux1 : Mux  Inputs=3
  Product{,1..8} (9 alike) : Product
  Uabc : Outport  VectorParamsAs1DForOutWhenUnconnected=off
  wires:
  pluse/1 -> Bus Selector/1
  Bus Selector/1 -> Product/2, Product/1  "<signal1>"
  Product/1 -> Add/1
  Bus Selector/2 -> Product1/2, Product1/1  "<signal2>"
  Product1/1 -> Add/2
  Bus Selector/3 -> Product2/2, Product2/1  "<signal3>"
  Product2/1 -> Add1/1
  Bus Selector/4 -> Product3/2, Product3/1  "<signal4>"
  Product3/1 -> Add1/2
  Bus Selector/5 -> Product4/2, Product4/1  "<signal5>"
  Product4/1 -> Add2/1
  Bus Selector/6 -> Product5/2, Product5/1  "<signal6>"
  Product5/1 -> Add2/2
  Add1/1 -> Mux/2
  Add/1 -> Mux/1
  Add2/1 -> Mux/3
  Mux/1 -> Fcn2/1, Fcn1/1, Fcn/1
  Fcn/1 -> Product6/2
  Fcn1/1 -> Product7/2
  Fcn2/1 -> Product8/2
  Product6/1 -> Mux1/1
  Product7/1 -> Mux1/2
  Product8/1 -> Mux1/3
  Constant/1 -> Product6/1, Product8/1, Product7/1
  Mux1/1 -> Uabc/1

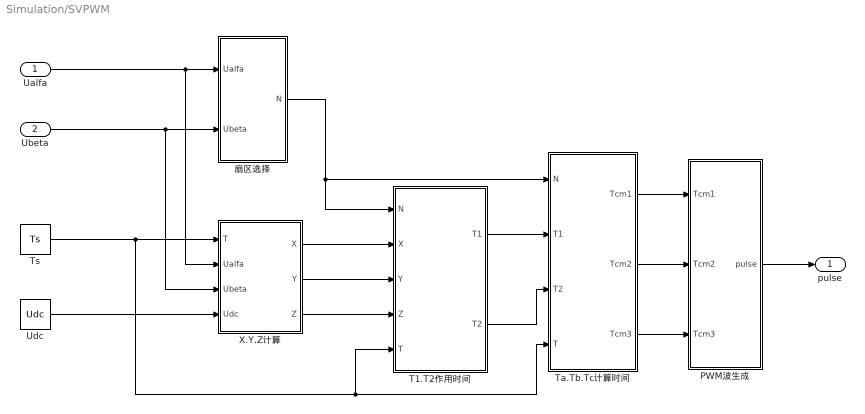
== system Simulation/SVPWM ==
  Ualfa : Inport
  Ubeta : Inport  Port=2
  " PWM波生成" : Subsystem
  T1.T2作用时间 : Subsystem
  Ta.Tb.Tc计算时间 : Subsystem
  Ts : Constant  Value=Ts  SampleTime=Tsc
  Udc : Constant  Value=Udc  SampleTime=Tsc
  X.Y.Z计算 : Subsystem
  扇区选择 : Subsystem
  pulse : Outport  VectorParamsAs1DForOutWhenUnconnected=off
  wires:
  " PWM波生成"/1(pulse) -> pulse/1
  Ubeta/1 -> X.Y.Z计算/3(Ubeta), 扇区选择/2(Ubeta)
  Ualfa/1 -> X.Y.Z计算/2(Ualfa), 扇区选择/1(Ualfa)
  Ta.Tb.Tc计算时间/3(Tcm3) -> " PWM波生成"/3(Tcm3)
  Ta.Tb.Tc计算时间/2(Tcm2) -> " PWM波生成"/2(Tcm2)
  Ta.Tb.Tc计算时间/1(Tcm1) -> " PWM波生成"/1(Tcm1)
  X.Y.Z计算/3(Z) -> T1.T2作用时间/4(Z)
  X.Y.Z计算/2(Y) -> T1.T2作用时间/3(Y)
  X.Y.Z计算/1(X) -> T1.T2作用时间/2(X)
  扇区选择/1(N) -> T1.T2作用时间/1(N), Ta.Tb.Tc计算时间/1(N)
  Udc/1 -> X.Y.Z计算/4(Udc)
  Ts/1 -> Ta.Tb.Tc计算时间/4(T), T1.T2作用时间/5(T), X.Y.Z计算/1(T)
  T1.T2作用时间/1(T1) -> Ta.Tb.Tc计算时间/2(T1)
  T1.T2作用时间/2(T2) -> Ta.Tb.Tc计算时间/3(T2)

== system Simulation/Subsystem1 ==
  abc : Inport  PortDimensions=3
  Demux : Demux  Outputs=3
  Gain12 : Gain  Gain="[ 1   -1/2   -1/2; 0   sqrt(3)/2   -sqrt(3)/2; 1/2  1/2  1/2 ]"  Multiplication=Matrix(K*u) (u vector)  SaturateOnIntegerOverflow=on  OutDataTypeStr=Inherit: Same as input  ParamDataTypeStr=Inherit: Same as input
  Gain4 : Gain  Gain=2/3  SaturateOnIntegerOverflow=on  OutDataTypeStr=Inherit: Same as input  ParamDataTypeStr=Inherit: Same as input
  Terminator : Terminator
  alpha : Outport  VectorParamsAs1DForOutWhenUnconnected=off
  beta : Outport  Port=2
  wires:
  Gain12/1 -> Gain4/1
  abc/1 -> Gain12/1
  Gain4/1 -> Demux/1
  Demux/1 -> alpha/1
  Demux/2 -> beta/1
  Demux/3 -> Terminator/1

== system Simulation/Subsystem10 ==
  abc : Inport  PortDimensions=3
  Demux : Demux  Outputs=3
  Gain12 : Gain  Gain="[ 1   -1/2   -1/2; 0   sqrt(3)/2   -sqrt(3)/2; 1/2  1/2  1/2 ]"  Multiplication=Matrix(K*u) (u vector)  SaturateOnIntegerOverflow=on  OutDataTypeStr=Inherit: Same as input  ParamDataTypeStr=Inherit: Same as input
  Gain4 : Gain  Gain=2/3  SaturateOnIntegerOverflow=on  OutDataTypeStr=Inherit: Same as input  ParamDataTypeStr=Inherit: Same as input
  Terminator : Terminator
  alpha : Outport  VectorParamsAs1DForOutWhenUnconnected=off
  beta : Outport  Port=2
  wires:
  Gain12/1 -> Gain4/1
  abc/1 -> Gain12/1
  Gain4/1 -> Demux/1
  Demux/1 -> alpha/1
  Demux/2 -> beta/1
  Demux/3 -> Terminator/1

== system Simulation/Subsystem2 ==
  abc : Inport  PortDimensions=3
  Demux : Demux  Outputs=3
  Gain12 : Gain  Gain="[ 1   -1/2   -1/2; 0   sqrt(3)/2   -sqrt(3)/2; 1/2  1/2  1/2 ]"  Multiplication=Matrix(K*u) (u vector)  SaturateOnIntegerOverflow=on  OutDataTypeStr=Inherit: Same as input  ParamDataTypeStr=Inherit: Same as input
  Gain4 : Gain  Gain=2/3  SaturateOnIntegerOverflow=on  OutDataTypeStr=Inherit: Same as input  ParamDataTypeStr=Inherit: Same as input
  Terminator : Terminator
  alpha : Outport  VectorParamsAs1DForOutWhenUnconnected=off
  beta : Outport  Port=2
  wires:
  Gain12/1 -> Gain4/1
  abc/1 -> Gain12/1
  Gain4/1 -> Demux/1
  Demux/1 -> alpha/1
  Demux/2 -> beta/1
  Demux/3 -> Terminator/1

== system Simulation/Subsystem3 ==
  abc : Inport  PortDimensions=3
  Demux : Demux  Outputs=3
  Gain12 : Gain  Gain="[ 1   -1/2   -1/2; 0   sqrt(3)/2   -sqrt(3)/2; 1/2  1/2  1/2 ]"  Multiplication=Matrix(K*u) (u vector)  SaturateOnIntegerOverflow=on  OutDataTypeStr=Inherit: Same as input  ParamDataTypeStr=Inherit: Same as input
  Gain4 : Gain  Gain=2/3  SaturateOnIntegerOverflow=on  OutDataTypeStr=Inherit: Same as input  ParamDataTypeStr=Inherit: Same as input
  Terminator : Terminator
  alpha : Outport  VectorParamsAs1DForOutWhenUnconnected=off
  beta : Outport  Port=2
  wires:
  Gain12/1 -> Gain4/1
  abc/1 -> Gain12/1
  Gain4/1 -> Demux/1
  Demux/1 -> alpha/1
  Demux/2 -> beta/1
  Demux/3 -> Terminator/1

== system Simulation/Subsystem4 ==
  note: d = al*cos(wt) + be*sin(wt)
  note: q = -al*sin(wt) + be*cos(wt)
  alpha : Inport
  beta : Inport  Port=2  PortDimensions=1
  wt : Inport  Port=3
  Fcn : Fcn  Expr=u(1)*cos(u(3)) + u(2)*sin(u(3))
  Fcn1 : Fcn  Expr=-u(1)*sin(u(3)) + u(2)*cos(u(3))
  Mux2 : Mux  Inputs=[1 1 1]
  d : Outport  InitialOutput=[0,0]  VectorParamsAs1DForOutWhenUnconnected=off
  q : Outport  Port=2
  wires:
  Fcn/1 -> d/1
  Mux2/1 -> Fcn1/1, Fcn/1
  Fcn1/1 -> q/1
  alpha/1 -> Mux2/1
  wt/1 -> Mux2/3
  beta/1 -> Mux2/2

== system Simulation/Subsystem5 ==
  d : Inport
  q : Inport  Port=2
  wt : Inport  Port=3  PortDimensions=1
  Fcn2 : Fcn  Expr=u(1)*cos(u(3)) - u(2)*sin(u(3))
  Fcn3 : Fcn  Expr=u(1)*sin(u(3)) + u(2)*cos(u(3))
  Mux2 : Mux  Inputs=[1 1 1]
  alpha : Outport  InitialOutput=[0,0]  VectorParamsAs1DForOutWhenUnconnected=off
  beta : Outport  Port=2
  wires:
  q/1 -> Mux2/2
  Mux2/1 -> Fcn2/1, Fcn3/1
  d/1 -> Mux2/1
  Fcn3/1 -> beta/1
  wt/1 -> Mux2/3
  Fcn2/1 -> alpha/1

== system Simulation/Subsystem6 ==
  note: d = al*cos(wt) + be*sin(wt)
  note: q = -al*sin(wt) + be*cos(wt)
  alpha : Inport
  beta : Inport  Port=2  PortDimensions=1
  wt : Inport  Port=3
  Fcn : Fcn  Expr=u(1)*cos(u(3)) + u(2)*sin(u(3))
  Fcn1 : Fcn  Expr=-u(1)*sin(u(3)) + u(2)*cos(u(3))
  Mux2 : Mux  Inputs=[1 1 1]
  d : Outport  InitialOutput=[0,0]  VectorParamsAs1DForOutWhenUnconnected=off
  q : Outport  Port=2
  wires:
  Fcn/1 -> d/1
  Mux2/1 -> Fcn1/1, Fcn/1
  Fcn1/1 -> q/1
  alpha/1 -> Mux2/1
  wt/1 -> Mux2/3
  beta/1 -> Mux2/2

== system Simulation/Subsystem7 ==
  abc : Inport  PortDimensions=3
  Demux : Demux  Outputs=3
  Gain12 : Gain  Gain="[ 1   -1/2   -1/2; 0   sqrt(3)/2   -sqrt(3)/2; 1/2  1/2  1/2 ]"  Multiplication=Matrix(K*u) (u vector)  SaturateOnIntegerOverflow=on  OutDataTypeStr=Inherit: Same as input  ParamDataTypeStr=Inherit: Same as input
  Gain4 : Gain  Gain=2/3  SaturateOnIntegerOverflow=on  OutDataTypeStr=Inherit: Same as input  ParamDataTypeStr=Inherit: Same as input
  Terminator : Terminator
  alpha : Outport  VectorParamsAs1DForOutWhenUnconnected=off
  beta : Outport  Port=2
  wires:
  Gain12/1 -> Gain4/1
  abc/1 -> Gain12/1
  Gain4/1 -> Demux/1
  Demux/1 -> alpha/1
  Demux/2 -> beta/1
  Demux/3 -> Terminator/1

== system Simulation/Subsystem8 ==
  d : Inport
  q : Inport  Port=2
  wt : Inport  Port=3  PortDimensions=1
  Fcn2 : Fcn  Expr=u(1)*cos(u(3)) - u(2)*sin(u(3))
  Fcn3 : Fcn  Expr=u(1)*sin(u(3)) + u(2)*cos(u(3))
  Mux2 : Mux  Inputs=[1 1 1]
  alpha : Outport  InitialOutput=[0,0]  VectorParamsAs1DForOutWhenUnconnected=off
  beta : Outport  Port=2
  wires:
  q/1 -> Mux2/2
  Mux2/1 -> Fcn2/1, Fcn3/1
  d/1 -> Mux2/1
  Fcn3/1 -> beta/1
  wt/1 -> Mux2/3
  Fcn2/1 -> alpha/1

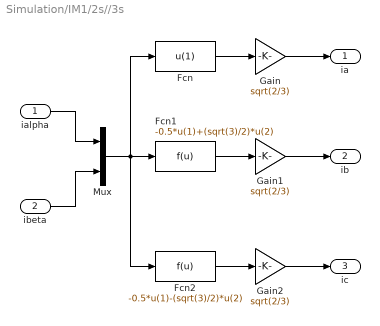
== system Simulation/IM1/2s//3s ==
  ialpha : Inport
  ibeta : Inport  Port=2
  Fcn : Fcn  Expr=u(1)
  Fcn1 : Fcn  Expr=-0.5*u(1)+(sqrt(3)/2)*u(2)
  Fcn2 : Fcn  Expr=-0.5*u(1)-(sqrt(3)/2)*u(2)
  Gain : Gain  Gain=sqrt(2/3)
  Gain1 : Gain  Gain=sqrt(2/3)
  Gain2 : Gain  Gain=sqrt(2/3)
  Mux : Mux  Inputs=2
  ia : Outport  VectorParamsAs1DForOutWhenUnconnected=off
  ib : Outport  Port=2  VectorParamsAs1DForOutWhenUnconnected=off
  ic : Outport  Port=3  VectorParamsAs1DForOutWhenUnconnected=off
  wires:
  ialpha/1 -> Mux/1
  ibeta/1 -> Mux/2
  Mux/1 -> Fcn2/1, Fcn1/1, Fcn/1
  Fcn/1 -> Gain/1
  Fcn1/1 -> Gain1/1
  Fcn2/1 -> Gain2/1
  Gain/1 -> ia/1
  Gain1/1 -> ib/1
  Gain2/1 -> ic/1

== system Simulation/IM1/3s//2s ==
  ua : Inport
  ub : Inport  Port=2
  uc : Inport  Port=3
  Fcn : Fcn  Expr=(u(1)-0.5*u(2)-0.5*u(3))*sqrt(2/3)
  Fcn1 : Fcn  Expr=(u(2)*(sqrt(3)/2)-u(3)*(sqrt(3)/2))*sqrt(2/3)
  Mux : Mux  Inputs=3
  ualpha : Outport  VectorParamsAs1DForOutWhenUnconnected=off
  ubeta : Outport  Port=2  VectorParamsAs1DForOutWhenUnconnected=off
  wires:
  ub/1 -> Mux/2
  ua/1 -> Mux/1
  uc/1 -> Mux/3
  Mux/1 -> Fcn1/1, Fcn/1
  Fcn/1 -> ualpha/1
  Fcn1/1 -> ubeta/1

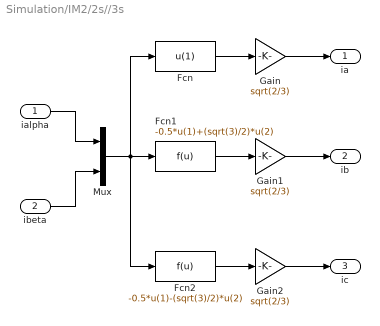
== system Simulation/IM2/2s//3s ==
  ialpha : Inport
  ibeta : Inport  Port=2
  Fcn : Fcn  Expr=u(1)
  Fcn1 : Fcn  Expr=-0.5*u(1)+(sqrt(3)/2)*u(2)
  Fcn2 : Fcn  Expr=-0.5*u(1)-(sqrt(3)/2)*u(2)
  Gain : Gain  Gain=sqrt(2/3)
  Gain1 : Gain  Gain=sqrt(2/3)
  Gain2 : Gain  Gain=sqrt(2/3)
  Mux : Mux  Inputs=2
  ia : Outport  VectorParamsAs1DForOutWhenUnconnected=off
  ib : Outport  Port=2  VectorParamsAs1DForOutWhenUnconnected=off
  ic : Outport  Port=3  VectorParamsAs1DForOutWhenUnconnected=off
  wires:
  ialpha/1 -> Mux/1
  ibeta/1 -> Mux/2
  Mux/1 -> Fcn2/1, Fcn1/1, Fcn/1
  Fcn/1 -> Gain/1
  Fcn1/1 -> Gain1/1
  Fcn2/1 -> Gain2/1
  Gain/1 -> ia/1
  Gain1/1 -> ib/1
  Gain2/1 -> ic/1

== system Simulation/IM2/3s//2s ==
  ua : Inport
  ub : Inport  Port=2
  uc : Inport  Port=3
  Fcn : Fcn  Expr=(u(1)-0.5*u(2)-0.5*u(3))*sqrt(2/3)
  Fcn1 : Fcn  Expr=(u(2)*(sqrt(3)/2)-u(3)*(sqrt(3)/2))*sqrt(2/3)
  Mux : Mux  Inputs=3
  ualpha : Outport  VectorParamsAs1DForOutWhenUnconnected=off
  ubeta : Outport  Port=2  VectorParamsAs1DForOutWhenUnconnected=off
  wires:
  ub/1 -> Mux/2
  ua/1 -> Mux/1
  uc/1 -> Mux/3
  Mux/1 -> Fcn1/1, Fcn/1
  Fcn/1 -> ualpha/1
  Fcn1/1 -> ubeta/1

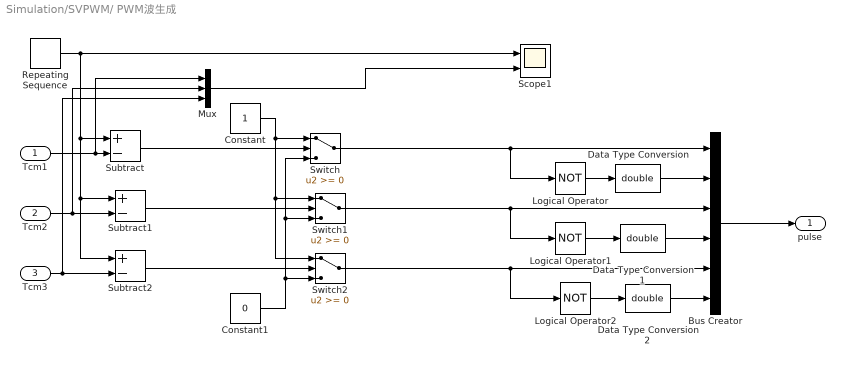
== system Simulation/SVPWM/ PWM波生成 ==
  Tcm1 : Inport
  Tcm2 : Inport  Port=2
  Tcm3 : Inport  Port=3
  Bus Creator : BusCreator  Inputs=6
  Constant : Constant
  Constant1 : Constant  Value=0
  Data Type Conversion : DataTypeConversion  OutDataTypeStr=double  SaturateOnIntegerOverflow=off  RndMeth=Floor
  Data Type Conversion1 : DataTypeConversion  OutDataTypeStr=double  SaturateOnIntegerOverflow=off  RndMeth=Floor
  Data Type Conversion2 : DataTypeConversion  OutDataTypeStr=double  SaturateOnIntegerOverflow=off  RndMeth=Floor
  Logical Operator : Logic  Operator=NOT  AllPortsSameDT=off
  Logical Operator1 : Logic  Operator=NOT  AllPortsSameDT=off
  Logical Operator2 : Logic  Operator=NOT  AllPortsSameDT=off
  Mux : Mux  Inputs=3
  Repeating Sequence : simulink/Sources/Repeating Sequence  rep_seq_t=[0 0.0001/2 0.0001]  rep_seq_y=[0 0.0001/2 0]
  Scope1 : Scope  NumInputPorts=2
  Subtract : Sum  Inputs=+-
  Subtract1 : Sum  Inputs=+-
  Subtract2 : Sum  Inputs=+-
  Switch : Switch  SaturateOnIntegerOverflow=off  InputSameDT=off
  Switch1 : Switch  SaturateOnIntegerOverflow=off  InputSameDT=off
  Switch2 : Switch  SaturateOnIntegerOverflow=off  InputSameDT=off
  pulse : Outport  VectorParamsAs1DForOutWhenUnconnected=off
  wires:
  Switch2/1 -> Logical Operator2/1, Bus Creator/5
  Switch/1 -> Logical Operator/1, Bus Creator/1
  Constant1/1 -> Switch2/3, Switch1/3, Switch/3
  Constant/1 -> Switch/1, Switch1/1, Switch2/1
  Data Type Conversion2/1 -> Bus Creator/6
  Data Type Conversion1/1 -> Bus Creator/4
  Data Type Conversion/1 -> Bus Creator/2
  Bus Creator/1 -> pulse/1
  Switch1/1 -> Logical Operator1/1, Bus Creator/3
  Logical Operator/1 -> Data Type Conversion/1
  Logical Operator2/1 -> Data Type Conversion2/1
  Logical Operator1/1 -> Data Type Conversion1/1
  Tcm3/1 -> Mux/3, Subtract2/2
  Tcm2/1 -> Mux/2, Subtract1/2
  Tcm1/1 -> Mux/1, Subtract/2
  Repeating Sequence/1 -> Scope1/1, Subtract1/1, Subtract2/1, Subtract/1
  Subtract2/1 -> Switch2/2
  Subtract1/1 -> Switch1/2
  Subtract/1 -> Switch/2
  Mux/1 -> Scope1/2

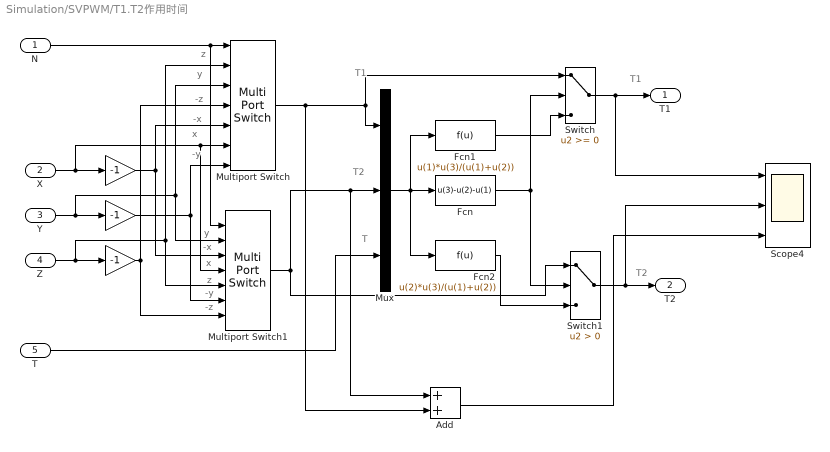
== system Simulation/SVPWM/T1.T2作用时间 ==
  note: T2
  note: T1
  note: T
  note: T2
  note: T1
  note: -z
  note: -y
  note: z
  note: x
  note: -x
  note: y
  note: -y
  note: x
  note: -x
  note: -z
  note: y
  note: z
  N : Inport
  X : Inport  Port=2
  Y : Inport  Port=3
  Z : Inport  Port=4
  T : Inport  Port=5
  " " : Gain  Gain=-1
  "  " : Gain  Gain=-1
  "    " : Gain  Gain=-1
  Add : Sum
  Fcn : Fcn  Expr=u(3)-u(2)-u(1)
  Fcn1 : Fcn  Expr=u(1)*u(3)/(u(1)+u(2))
  Fcn2 : Fcn  Expr=u(2)*u(3)/(u(1)+u(2))
  Multiport Switch : MultiPortSwitch  Inputs=6  SaturateOnIntegerOverflow=off  InputSameDT=off
  Multiport Switch1 : MultiPortSwitch  Inputs=6  SaturateOnIntegerOverflow=off  InputSameDT=off
  Mux : Mux  Inputs=3
  Scope4 : Scope  NumInputPorts=3
  Switch : Switch  SaturateOnIntegerOverflow=off  InputSameDT=off
  Switch1 : Switch  Criteria=u2 > Threshold  SaturateOnIntegerOverflow=off  InputSameDT=off
  T1 : Outport  VectorParamsAs1DForOutWhenUnconnected=off
  T2 : Outport  Port=2  VectorParamsAs1DForOutWhenUnconnected=off
  wires:
  Add/1 -> Scope4/3
  Switch1/1 -> Scope4/2, T2/1
  Switch/1 -> Scope4/1, T1/1
  Fcn2/1 -> Switch1/3
  Fcn1/1 -> Switch/3
  Fcn/1 -> Switch1/2, Switch/2
  Mux/1 -> Fcn2/1, Fcn1/1, Fcn/1
  T/1 -> Mux/3
  Multiport Switch1/1 -> Add/1, Mux/2, Switch1/1
  Multiport Switch/1 -> Add/2, Switch/1, Mux/1
  " "/1 -> Multiport Switch1/3, Multiport Switch/5
  "  "/1 -> Multiport Switch1/6, Multiport Switch/7
  "    "/1 -> Multiport Switch/4, Multiport Switch1/7
  Z/1 -> "    "/1, Multiport Switch/2, Multiport Switch1/5
  Y/1 -> "  "/1, Multiport Switch/3, Multiport Switch1/2
  X/1 -> " "/1, Multiport Switch/6, Multiport Switch1/4
  N/1 -> Multiport Switch/1, Multiport Switch1/1

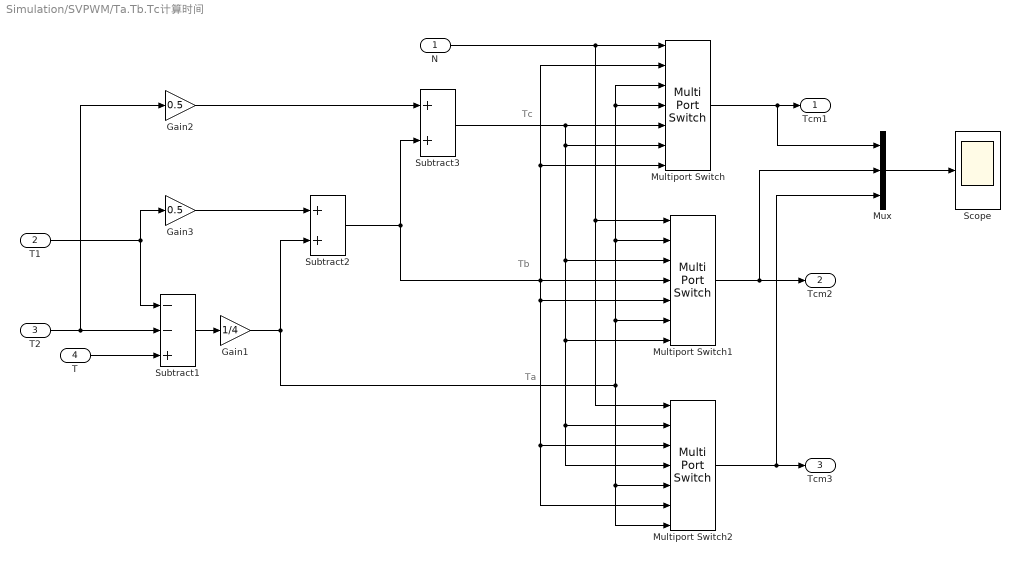
== system Simulation/SVPWM/Ta.Tb.Tc计算时间 ==
  note: Ta
  note: Tb
  note: Tc
  N : Inport
  T1 : Inport  Port=2
  T2 : Inport  Port=3
  T : Inport  Port=4
  Gain1 : Gain  Gain=1/4
  Gain2 : Gain  Gain=0.5
  Gain3 : Gain  Gain=0.5
  Multiport Switch : MultiPortSwitch  Inputs=6  SaturateOnIntegerOverflow=off  InputSameDT=off
  Multiport Switch1 : MultiPortSwitch  Inputs=6  SaturateOnIntegerOverflow=off  InputSameDT=off
  Multiport Switch2 : MultiPortSwitch  Inputs=6  SaturateOnIntegerOverflow=off  InputSameDT=off
  Mux : Mux  Inputs=3
  Scope : Scope
  Subtract1 : Sum  Inputs=--+
  Subtract2 : Sum
  Subtract3 : Sum
  Tcm1 : Outport  VectorParamsAs1DForOutWhenUnconnected=off
  Tcm2 : Outport  Port=2  VectorParamsAs1DForOutWhenUnconnected=off
  Tcm3 : Outport  Port=3  VectorParamsAs1DForOutWhenUnconnected=off
  wires:
  Subtract3/1 -> Multiport Switch2/4, Multiport Switch2/2, Multiport Switch1/7, Multiport Switch1/3, Multiport Switch/6, Multiport Switch/5
  Multiport Switch2/1 -> Mux/3, Tcm3/1
  Multiport Switch1/1 -> Mux/2, Tcm2/1
  Multiport Switch/1 -> Mux/1, Tcm1/1
  N/1 -> Multiport Switch1/1, Multiport Switch2/1, Multiport Switch/1
  Gain2/1 -> Subtract3/1
  Subtract2/1 -> Multiport Switch/7, Multiport Switch/2, Multiport Switch2/6, Multiport Switch2/3, Multiport Switch1/5, Multiport Switch1/4, Subtract3/2
  Gain1/1 -> Subtract2/2, Multiport Switch1/6, Multiport Switch1/2, Multiport Switch/4, Multiport Switch/3, Multiport Switch2/7, Multiport Switch2/5
  Subtract1/1 -> Gain1/1
  Gain3/1 -> Subtract2/1
  T1/1 -> Subtract1/1, Gain3/1
  T/1 -> Subtract1/3
  T2/1 -> Subtract1/2, Gain2/1
  Mux/1 -> Scope/1

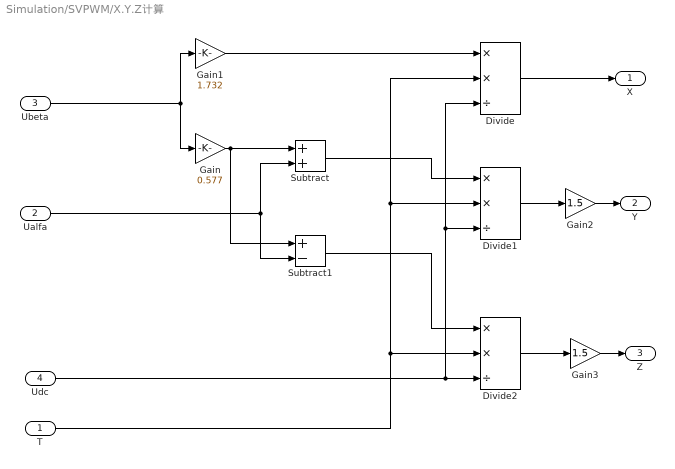
== system Simulation/SVPWM/X.Y.Z计算 ==
  T : Inport
  Ualfa : Inport  Port=2
  Ubeta : Inport  Port=3
  Udc : Inport  Port=4
  Divide : Product  Inputs=**/
  Divide1 : Product  Inputs=**/
  Divide2 : Product  Inputs=**/
  Gain : Gain  Gain=0.577
  Gain1 : Gain  Gain=1.732
  Gain2 : Gain  Gain=1.5
  Gain3 : Gain  Gain=1.5
  Subtract : Sum
  Subtract1 : Sum  Inputs=+-
  X : Outport  VectorParamsAs1DForOutWhenUnconnected=off
  Y : Outport  Port=2  VectorParamsAs1DForOutWhenUnconnected=off
  Z : Outport  Port=3  VectorParamsAs1DForOutWhenUnconnected=off
  wires:
  Ubeta/1 -> Gain/1, Gain1/1
  Gain3/1 -> Z/1
  Gain2/1 -> Y/1
  Divide2/1 -> Gain3/1
  Divide1/1 -> Gain2/1
  Divide/1 -> X/1
  Subtract1/1 -> Divide2/1
  Subtract/1 -> Divide1/1
  Ualfa/1 -> Subtract/2, Subtract1/2
  Udc/1 -> Divide/3, Divide1/3, Divide2/3
  T/1 -> Divide/2, Divide1/2, Divide2/2
  Gain1/1 -> Divide/1
  Gain/1 -> Subtract1/1, Subtract/1

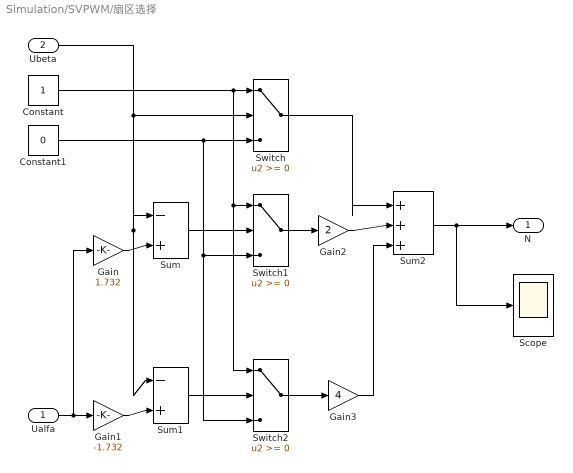
== system Simulation/SVPWM/扇区选择 ==
  Ualfa : Inport
  Ubeta : Inport  Port=2
  Constant : Constant
  Constant1 : Constant  Value=0
  Gain : Gain  Gain=1.732
  Gain1 : Gain  Gain=-1.732
  Gain2 : Gain  Gain=2
  Gain3 : Gain  Gain=4
  Scope : Scope
  Sum : Sum  Inputs=|-+
  Sum1 : Sum  Inputs=|-+
  Sum2 : Sum  Inputs=|+++
  Switch : Switch  SaturateOnIntegerOverflow=off  InputSameDT=off
  Switch1 : Switch  SaturateOnIntegerOverflow=off  InputSameDT=off
  Switch2 : Switch  SaturateOnIntegerOverflow=off  InputSameDT=off
  N : Outport  VectorParamsAs1DForOutWhenUnconnected=off
  wires:
  Sum2/1 -> Scope/1, N/1
  Gain3/1 -> Sum2/3
  Switch/1 -> Sum2/1
  Gain2/1 -> Sum2/2
  Switch2/1 -> Gain3/1
  Switch1/1 -> Gain2/1
  Constant1/1 -> Switch2/3, Switch1/3, Switch/3
  Gain1/1 -> Sum1/2
  Sum1/1 -> Switch2/2
  Sum/1 -> Switch1/2
  Gain/1 -> Sum/2
  Ualfa/1 -> Gain/1, Gain1/1
  Constant/1 -> Switch1/1, Switch2/1, Switch/1
  Ubeta/1 -> Sum1/1, Sum/1, Switch/2
